simulink model "EEE4022S_Single_Pendulum_SIM"  (R2021a)
settings: Solver=ode4  StartTime=0.0  StopTime=60  FixedStep=0.002  RelTol=1e-3
values from neighbouring files (symbols this model uses):
  A = [cos(th)   sin(th) 0;          -sin(th)  cos(th) 0;          0        0        1]    [EEE4022S_Single_Pendulum.m]
  B = double(B)    [EEE4022S_Single_Pendulum.m]
  C1 = [ ... (first row only)    [EEE4022S_Single_Pendulum.m]
  D = [ ... (first row only)    [EEE4022S_Single_Pendulum.m]
  g = 9.81    [EEE4022S_Single_Pendulum.m]
  J = 0.0073    [EEE4022S_Single_Pendulum.m]
  K = lqr(A,B,Q,R)    [EEE4022S_Single_Pendulum.m]
  l = 0.3302    [EEE4022S_Single_Pendulum.m]
  mp = 0.230    (= 0.23)    [EEE4022S_Single_Pendulum.m]
  wcf = 2 * pi * 10.0    (= 62.8318530718)    [EEE4022S_Single_Pendulum.m]
  zetaf = 0.9    [EEE4022S_Single_Pendulum.m]
libraries: simulink x4, simulink_extras x3
settings Model: Creator=User  LastModifiedBy=User
settings SolverCC: AutoInsertRateTranBlk=on

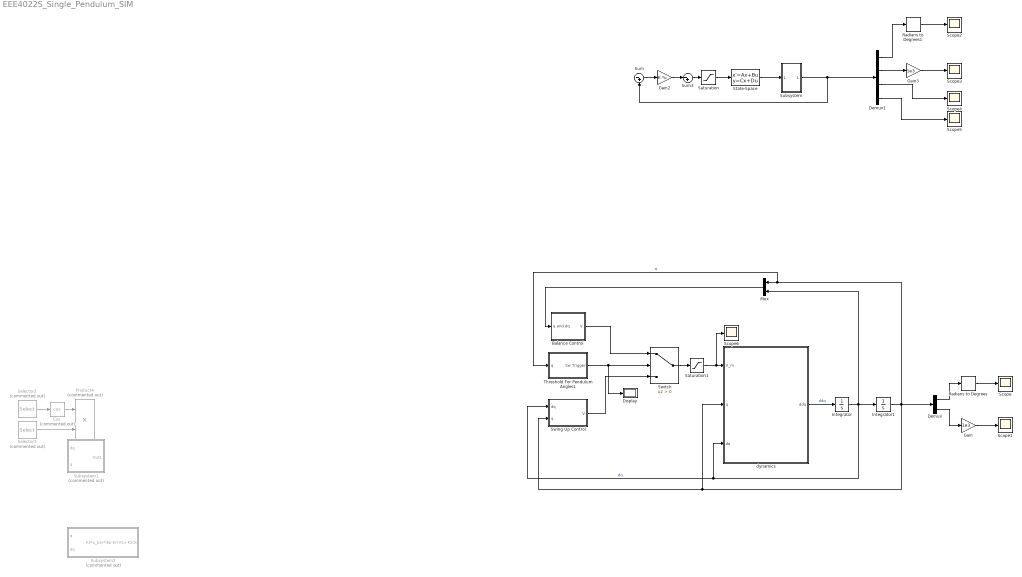
== system EEE4022S_Single_Pendulum_SIM ==
  Balance Control : Subsystem
  Cos : Trigonometry  Commented=on  Operator=cos
  Demux : Demux  Outputs=2
  Demux1 : Demux
  Display : Display
  Gain : Gain  Gain=1e3
  Gain2 : Gain  Gain=K  Multiplication=Matrix(K*u)
  Gain3 : Gain  Gain=1e3
  Integrator : Integrator  InitialCondition=[0 0]
  Integrator1 : Integrator  InitialCondition=[5*pi/180 0]
  Mux : Mux  Inputs=2
  Product4 : Product  Commented=on
  Radians to Degrees : simulink_extras/Transformations/Radians to Degrees
  Radians to Degrees1 : simulink_extras/Transformations/Radians to Degrees
  Saturation : Saturate  UpperLimit=24  LowerLimit=-24
  Saturation1 : Saturate  UpperLimit=24  LowerLimit=-24
  Scope{,1..6} (7 alike) : Scope
  Selector2 : Selector  Commented=on  InputPortWidth=2  IndexOptions=Index vector (dialog)  Indices=[1]  OutputSizes=1
  Selector3 : Selector  Commented=on  InputPortWidth=2  IndexOptions=Index vector (dialog)  Indices=[1]  OutputSizes=1
  State-Space : StateSpace  A=A  B=B  C=C1  D=D  InitialCondition=[45*pi/180 0 0 0]
  Subsystem : Subsystem
  Subsystem1 : Subsystem  Commented=on
  Subsystem2 : Subsystem  Commented=on
  Sum : Sum  Inputs=|-+
  Sum3 : Sum  Inputs=|-+
  Swing Up Control : Subsystem
  Switch : Switch  Criteria=u2 > Threshold
  Threshold For Pendulum Angles1 : Subsystem
  dynamics : MATLAB Function  TreatAsAtomicUnit=on
  wires:
  dynamics/1(ddq) -> Integrator/1  "ddq"
  Integrator/1 -> Swing Up Control/1(dq), dynamics/3(dq), Mux/2, Integrator1/1  "dq"
  Integrator1/1 -> Swing Up Control/2(q), dynamics/2(q), Threshold For Pendulum Angles1/1(q), Mux/1, Demux/1  "q"
  Demux/2 -> Gain/1
  Demux/1 -> Radians to Degrees/1
  Radians to Degrees/1 -> Scope/1
  Gain/1 -> Scope1/1
  Subsystem/1(Out1) -> Demux1/1, Sum/2
  Sum/1 -> Gain2/1
  Demux1/1 -> Radians to Degrees1/1
  Radians to Degrees1/1 -> Scope2/1
  Demux1/2 -> Gain3/1
  Gain3/1 -> Scope3/1
  State-Space/1 -> Subsystem/1(In1)
  Switch/1 -> Saturation1/1
  Demux1/3 -> Scope4/1
  Demux1/4 -> Scope5/1
  Gain2/1 -> Sum3/1
  Saturation/1 -> State-Space/1
  Sum3/1 -> Saturation/1
  Mux/1 -> Balance Control/1(q and dq)
  Balance Control/1(V) -> Switch/1
  Threshold For Pendulum Angles1/1(Sw Trigger) -> Display/1, Switch/2
  Saturation1/1 -> Scope6/1, dynamics/1(V_m)
  Cos/1 -> Product4/1
  Selector2/1 -> Cos/1
  Selector3/1 -> Product4/2
  Swing Up Control/1(V) -> Switch/3

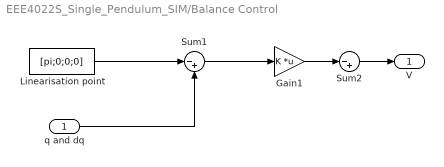
== system EEE4022S_Single_Pendulum_SIM/Balance Control ==
  q and dq : Inport
  Gain1 : Gain  Gain=K  Multiplication=Matrix(K*u)
  Linearisation point : Constant  Value=[pi;0;0;0]
  Sum1 : Sum  Inputs=|-+
  Sum2 : Sum  Inputs=|-+
  V : Outport
  wires:
  q and dq/1 -> Sum1/2
  Sum1/1 -> Gain1/1
  Linearisation point/1 -> Sum1/1
  Gain1/1 -> Sum2/1
  Sum2/1 -> V/1

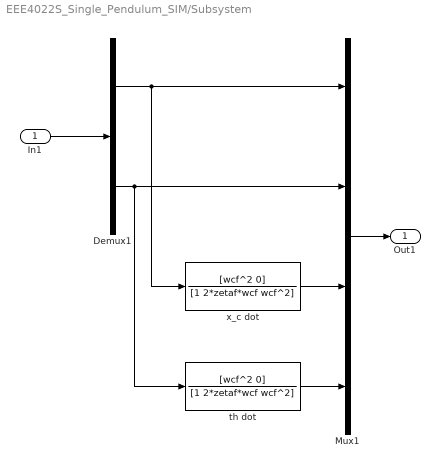
== system EEE4022S_Single_Pendulum_SIM/Subsystem ==
  In1 : Inport
  Demux1 : Demux  Outputs=2
  Mux1 : Mux
  th dot : TransferFcn  Numerator=[wcf^2 0]  Denominator=[1 2*zetaf*wcf wcf^2]
  x_c dot : TransferFcn  Numerator=[wcf^2 0]  Denominator=[1 2*zetaf*wcf wcf^2]
  Out1 : Outport
  wires:
  In1/1 -> Demux1/1
  Mux1/1 -> Out1/1
  Demux1/1 -> x_c dot/1, Mux1/1
  x_c dot/1 -> Mux1/3
  Demux1/2 -> th dot/1, Mux1/2
  th dot/1 -> Mux1/4

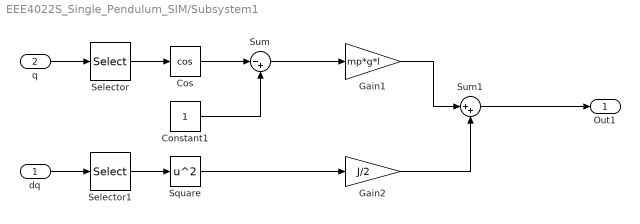
== system EEE4022S_Single_Pendulum_SIM/Subsystem1 ==
  dq : Inport
  q : Inport  Port=2
  Constant1 : Constant
  Cos : Trigonometry  Operator=cos
  Gain1 : Gain  Gain=mp*g*l
  Gain2 : Gain  Gain=J/2
  Selector : Selector  InputPortWidth=2  IndexOptions=Index vector (dialog)  Indices=[1]  OutputSizes=1
  Selector1 : Selector  InputPortWidth=2  IndexOptions=Index vector (dialog)  Indices=[1]  OutputSizes=1
  Square : Math  Operator=square  SaturateOnIntegerOverflow=on
  Sum : Sum  Inputs=|-+
  Sum1 : Sum  Inputs=|++
  Out1 : Outport
  wires:
  dq/1 -> Selector1/1
  Gain1/1 -> Sum1/1
  Sum/1 -> Gain1/1
  Sum1/1 -> Out1/1
  Constant1/1 -> Sum/2
  q/1 -> Selector/1
  Gain2/1 -> Sum1/2
  Square/1 -> Gain2/1
  Cos/1 -> Sum/1
  Selector/1 -> Cos/1
  Selector1/1 -> Square/1

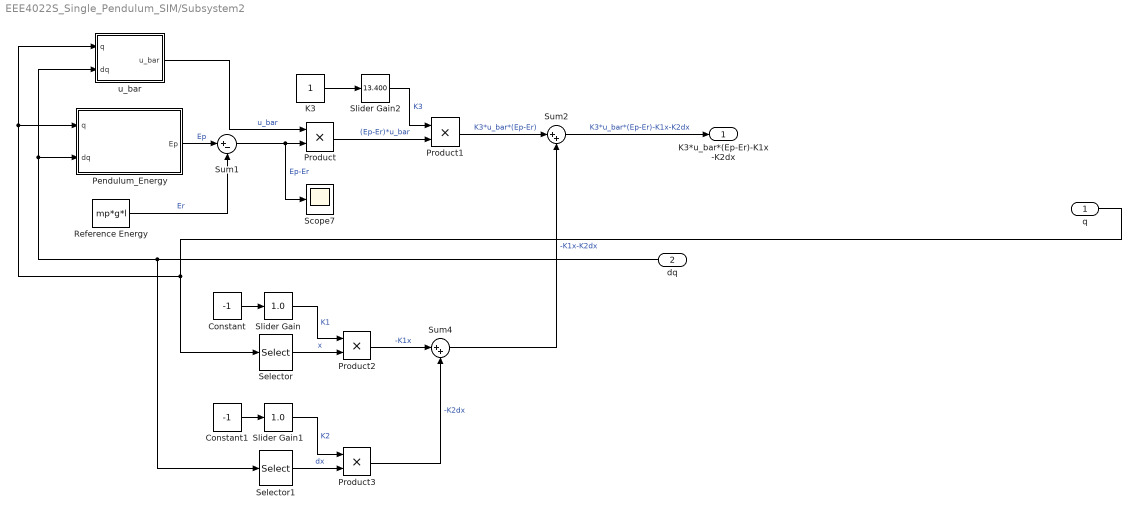
== system EEE4022S_Single_Pendulum_SIM/Subsystem2 ==
  q : Inport
  dq : Inport  Port=2
  Constant : Constant  Value=-1
  Constant1 : Constant  Value=-1
  K3 : Constant
  Pendulum_Energy : MATLAB Function  TreatAsAtomicUnit=on
  Product{,1..3} (4 alike) : Product
  Reference Energy : Constant  Value=mp*g*l
  Scope7 : Scope
  Selector : Selector  InputPortWidth=2  IndexOptions=Index vector (dialog)  Indices=[2]  OutputSizes=1
  Selector1 : Selector  InputPortWidth=2  IndexOptions=Index vector (dialog)  Indices=[2]  OutputSizes=1
  Slider Gain : simulink/Math Operations/Slider Gain  gain=1.0  low=0  high=20
  Slider Gain1 : simulink/Math Operations/Slider Gain  gain=1.0  low=0  high=20
  Slider Gain2 : simulink/Math Operations/Slider Gain  gain=13.400  low=0  high=20
  Sum1 : Sum  Inputs=|+-
  Sum2 : Sum  Inputs=|++
  Sum4 : Sum  Inputs=|++
  u_bar : MATLAB Function  TreatAsAtomicUnit=on
  K3*u_bar*(Ep-Er)-K1x-K2dx : Outport
  wires:
  Product1/1 -> Sum2/1  "K3*u_bar*(Ep-Er)"
  Sum4/1 -> Sum2/2  "-K1x-K2dx"
  dq/1 -> Selector1/1, Pendulum_Energy/2(dq), u_bar/2(dq)
  Constant1/1 -> Slider Gain1/1
  Sum1/1 -> Scope7/1, Product/2  "Ep-Er"
  Slider Gain/1 -> Product2/1  "K1"
  K3/1 -> Slider Gain2/1
  Pendulum_Energy/1(Ep) -> Sum1/1  "Ep"
  u_bar/1(u_bar) -> Product/1  "u_bar"
  Reference Energy/1 -> Sum1/2  "Er"
  Selector/1 -> Product2/2  "x"
  q/1 -> Selector/1, Pendulum_Energy/1(q), u_bar/1(q)
  Slider Gain2/1 -> Product1/1  "K3"
  Constant/1 -> Slider Gain/1
  Slider Gain1/1 -> Product3/1  "K2"
  Product2/1 -> Sum4/1  "-K1x"
  Selector1/1 -> Product3/2  "dx"
  Product/1 -> Product1/2  "(Ep-Er)*u_bar"
  Product3/1 -> Sum4/2  "-K2dx"
  Sum2/1 -> K3*u_bar*(Ep-Er)-K1x-K2dx/1  "K3*u_bar*(Ep-Er)-K1x-K2dx"

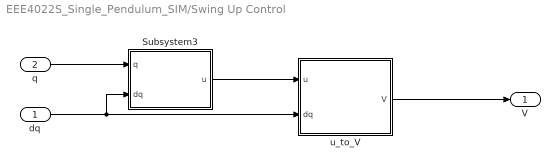
== system EEE4022S_Single_Pendulum_SIM/Swing Up Control ==
  dq : Inport
  q : Inport  Port=2
  Subsystem3 : Subsystem
  u_to_V : MATLAB Function  TreatAsAtomicUnit=on
  V : Outport
  wires:
  Subsystem3/1(u) -> u_to_V/1(u)
  dq/1 -> u_to_V/2(dq), Subsystem3/2(dq)
  u_to_V/1(V) -> V/1
  q/1 -> Subsystem3/1(q)

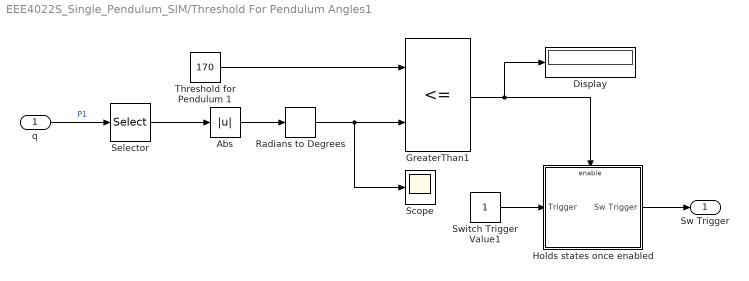
== system EEE4022S_Single_Pendulum_SIM/Threshold For Pendulum Angles1 ==
  q : Inport
  Abs : Abs
  Display : Display
  GreaterThan1 : RelationalOperator  Operator=<=  OutDataTypeStr=boolean  RndMeth=Simplest
  Holds states once enabled : Subsystem  TreatAsAtomicUnit=on
  Radians to Degrees : simulink_extras/Transformations/Radians to Degrees
  Scope : Scope
  Selector : Selector  InputPortWidth=2  IndexOptions=Index vector (dialog)  Indices=[1]  OutputSizes=1
  Switch Trigger Value1 : Constant
  Threshold for Pendulum 1 : Constant  Value=170
  Sw Trigger : Outport
  wires:
  GreaterThan1/1 -> Holds states once enabled/Enable, Display/1
  Holds states once enabled/1(Sw Trigger) -> Sw Trigger/1
  Switch Trigger Value1/1 -> Holds states once enabled/1(Trigger)
  q/1 -> Selector/1  "P1"
  Threshold for Pendulum 1/1 -> GreaterThan1/1
  Abs/1 -> Radians to Degrees/1
  Selector/1 -> Abs/1
  Radians to Degrees/1 -> Scope/1, GreaterThan1/2

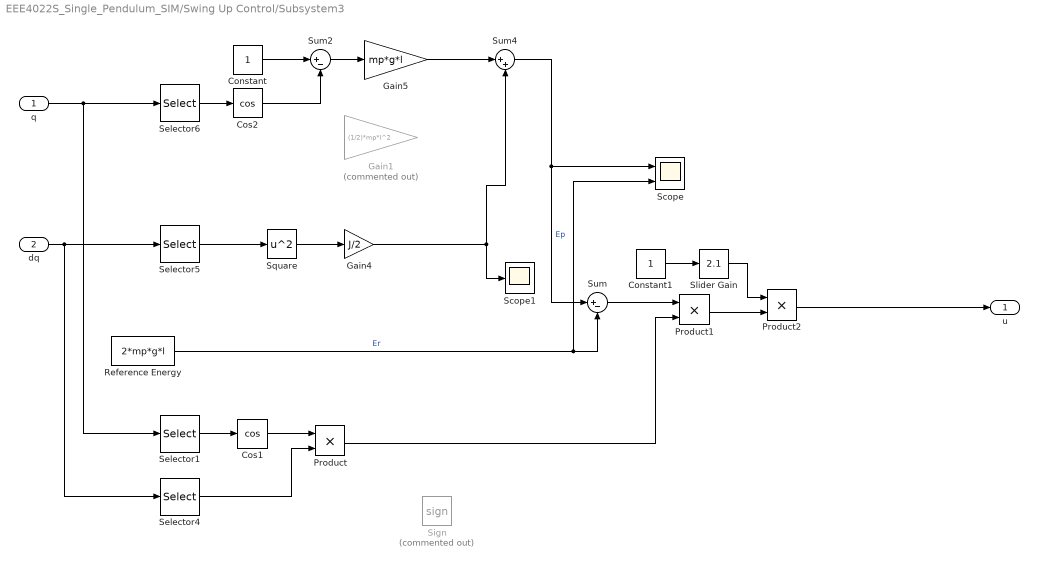
== system EEE4022S_Single_Pendulum_SIM/Swing Up Control/Subsystem3 ==
  q : Inport
  dq : Inport  Port=2
  Constant : Constant
  Constant1 : Constant
  Cos1 : Trigonometry  Operator=cos
  Cos2 : Trigonometry  Operator=cos
  Gain1 : Gain  Commented=on  Gain=(1/2)*mp*l^2
  Gain4 : Gain  Gain=J/2
  Gain5 : Gain  Gain=mp*g*l
  Product : Product
  Product1 : Product
  Product2 : Product
  Reference Energy : Constant  Value=2*mp*g*l
  Scope : Scope  NumInputPorts=2
  Scope1 : Scope
  Selector{1,4..6} (4 alike) : Selector  InputPortWidth=2  IndexOptions=Index vector (dialog)  Indices=[1]  OutputSizes=1
  Sign : Signum  Commented=on
  Slider Gain : simulink/Math Operations/Slider Gain  gain=2.1  low=0  high=10
  Square : Math  Operator=square  SaturateOnIntegerOverflow=on
  Sum : Sum  Inputs=|+-
  Sum2 : Sum  Inputs=|+-
  Sum4 : Sum  Inputs=|++
  u : Outport
  wires:
  Gain5/1 -> Sum4/1
  Product1/1 -> Product2/2
  Gain4/1 -> Sum4/2, Scope1/1
  Selector6/1 -> Cos2/1
  Selector4/1 -> Product/2
  Sum2/1 -> Gain5/1
  Cos1/1 -> Product/1
  Slider Gain/1 -> Product2/1
  Constant/1 -> Sum2/1
  Selector5/1 -> Square/1
  Cos2/1 -> Sum2/2
  Constant1/1 -> Slider Gain/1
  Selector1/1 -> Cos1/1
  Reference Energy/1 -> Scope/2, Sum/2  "Er"
  dq/1 -> Selector4/1, Selector5/1
  q/1 -> Selector1/1, Selector6/1
  Sum4/1 -> Sum/1, Scope/1  "Ep"
  Sum/1 -> Product1/1
  Product/1 -> Product1/2
  Square/1 -> Gain4/1
  Product2/1 -> u/1

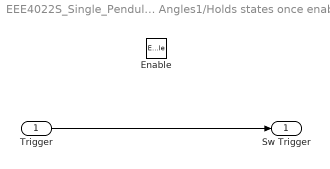
== system EEE4022S_Single_Pendulum_SIM/Threshold For Pendulum Angles1/Holds states once enabled ==
  Trigger : Inport  OutDataTypeStr=double
  Enable : EnablePort
  Sw Trigger : Outport  OutDataTypeStr=double  InitialOutput=[0]
  wires:
  Trigger/1 -> Sw Trigger/1

== matlab function EEE4022S_Single_Pendulum_SIM/Subsystem2/Pendulum_Energy ==
  data: q input; Ep output; dq input
function Ep = Pendulum_Energy(q,dq)
%#codegen

%    This function was generated by the Symbolic Math Toolbox version 8.7.
%    25-Oct-2022 17:45:25

th = q(1);
dth = dq(1);

g = 9.81;
mp = 0.230;
l = 0.3302;
J = 0.0073;

t2 = dth.^2;
Ep = (J.*t2)./2.0+(l.^2.*mp.*t2)./2.0-g.*l.*mp.*cos(th);

== matlab function EEE4022S_Single_Pendulum_SIM/dynamics ==
  data: ddq output; V_m input; q input; dq input
function ddq = dynamics(V_m,q,dq)
%#codegen

%    This function was generated by the Symbolic Math Toolbox version 8.7.
%    25-Oct-2022 12:32:13

th = q(1);
dth = dq(1);
dx = dq(2);

g = 9.81;
mp = 0.230;
mc = 0.57;
l = 0.3302;
Bc = 9.3378;
Bp = 0.0019;
J = 0.0073;

R_m = 2.6; 
k_t = 0.00767;
n_m = 1;
k_m = 0.00767;
K_g = 3.71;
n_g = 1;
r_mp = 6.35*10^(-3);

t2 = cos(th);
t3 = sin(th);
t4 = J.*mc;
t5 = J.*mp;
t6 = K_g.^2;
t7 = dth.^2;
t8 = l.^2;
t9 = mp.^2;
t10 = r_mp.^2;
t12 = 1.0./R_m;
t11 = t2.^2;
t13 = 1.0./t10;
t14 = mc.*mp.*t8;
t15 = t8.*t9;
t16 = t11.*t15;
t17 = -t16;
t18 = t4+t5+t14+t15+t17;
t19 = 1.0./t18;
ddq = [-t12.*t13.*t19.*(Bp.*R_m.*dth.*mc.*t10+Bp.*R_m.*dth.*mp.*t10+R_m.*g.*l.*t3.*t9.*t10+R_m.*t2.*t3.*t7.*t10.*t15-Bc.*R_m.*dx.*l.*mp.*t2.*t10+R_m.*g.*l.*mc.*mp.*t3.*t10+K_g.*V_m.*k_t.*l.*mp.*n_g.*n_m.*r_mp.*t2-dx.*k_m.*k_t.*l.*mp.*n_g.*n_m.*t2.*t6);t12.*t13.*t19.*(-Bc.*J.*R_m.*dx.*t10+(R_m.*g.*t10.*t15.*sin(th.*2.0))./2.0+R_m.*l.^3.*t3.*t7.*t9.*t10-Bc.*R_m.*dx.*mp.*t8.*t10+R_m.*l.*t3.*t5.*t7.*t10+J.*K_g.*V_m.*k_t.*n_g.*n_m.*r_mp+Bp.*R_m.*dth.*l.*mp.*t2.*t10-J.*dx.*k_m.*k_t.*n_g.*n_m.*t6+K_g.*V_m.*k_t.*mp.*n_g.*n_m.*r_mp.*t8-dx.*k_m.*k_t.*mp.*n_g.*n_m.*t6.*t8)];

== matlab function EEE4022S_Single_Pendulum_SIM/Subsystem2/u_bar ==
  data: q input; u_bar output; dq input
function u_bar = u_bar(q,dq)
%#codegen

%    This function was generated by the Symbolic Math Toolbox version 8.7.

th = q(1);
dth = dq(1);

mp = 0.230;
l = 0.3302;

u_bar = dth.*l.*mp.*cos(th);

== matlab function EEE4022S_Single_Pendulum_SIM/Swing Up Control/u_to_V ==
  data: u input; dq input; V output
function V = u_to_V(u,dq)
%#codegen

%    This function was generated by the Symbolic Math Toolbox version 8.7.
%    26-Oct-2022 11:43:40

dx = dq(2);

mc = 0.57;

R_m = 2.6; 
k_t = 0.00767;
n_m = 1;
k_m = 0.00767;
K_g = 3.71;
n_g = 1;
r_mp = 6.35*10^(-3);

V = (K_g.*dx.*k_m)./r_mp+(R_m.*mc.*r_mp.*u)./(K_g.*k_t.*n_g.*n_m);
